simulink model "Mission__SimulatorModel"  (Simulink 10.1)
settings: Solver=ode8  StartTime=0.0  StopTime=100000  FixedStep=time_step  RelTol=1e-3
StartFcn:
  | % copyfile(char(CurrentFolder + "\3DModels\" + string(MODELO_3D)), char(CurrentFolder + "\" + string(MODELO_3D)));
StopFcn:
  | % delete(MODELO_3D)
values from neighbouring files (symbols this model uses):
  Aileron_Trim = -deltaa_trim_med/2    [Trim_ArcDME2.m]
  Elevator_Trim = deltae_trim_med    [Trim_ArcDME2.m]    (also in Trim_ClimbXZ2.m; Trim_CruiseThetaXZ2.m)
  Engine_Trim = lever_trim_med    [Trim_ArcDME2.m]    (also in Trim_ClimbXZ2.m; Trim_CruiseThetaXZ2.m)
  phi_ini = phi_ini_trim_med    [Trim_ArcDME2.m]
  u_ini = u_ini_trim_med    [Trim_ArcDME2.m]    (also in Trim_ClimbXZ2.m; Trim_CruiseThetaXZ2.m)
  v_ini = v_ini_trim2    [Trim_ArcDME2.m]    (also in Trim_ClimbXZ2.m; Trim_CruiseThetaXZ2.m)
  w_ini = -UVW_aux(3)    [Trim_ArcDME2.m]    (also in Trim_ClimbXZ2.m = -UVW_aux2(3) + UVW_aux1(3); Trim_CruiseThetaXZ2.m)
undefined symbols (not defined in the file or in its folder): AoA_alpha_max, AoA_beta_max, b, c, cargo_mass, CD0_interp, CD_ajus_coef, CD_beta_interp, CD_mach_reg, CDde, CDflap, CDgear, CDi, CDsb, CDsp, CL_ajus_coef, CL_alpha_interp, CL_alpha_reg, Clb, Clda_interp, CLde, Cldr, Clp, Clr, Cm0, Cm_alpha, Cmadot, Cmde_ajus_coef, Cmde_interp, Cmq, Cnb, Cndr, Cnr, Coef_Aileron_Beta, Coef_Aileron_Phi, Coef_Aileron_Rudder, Coef_Elevator_Alpha, Coef_Rudder_Aileron, Coef_Rudder_Beta, CYb, dCLflap, dfuel, dfuel0, e0_0, e1_0, e2_0, e3_0, fuel, fuel_density, fuel_max, g, GeoDate_Ap, GeoDate_Day, GeoDate_LatLongElv, GeoDate_Time, Ixx, Ixz, Iyy, Izz, kCDge_interp ... (+35)
libraries: aerolibconvert2 x17, aerolibutil x14, dsppolyfun x7, aerolibactuator x5, sharedtransform x4, robotcorelib x4, simulink x3, visionstatistics x3, vrlib x2, aerolibasang x1
(part 2 of 3)

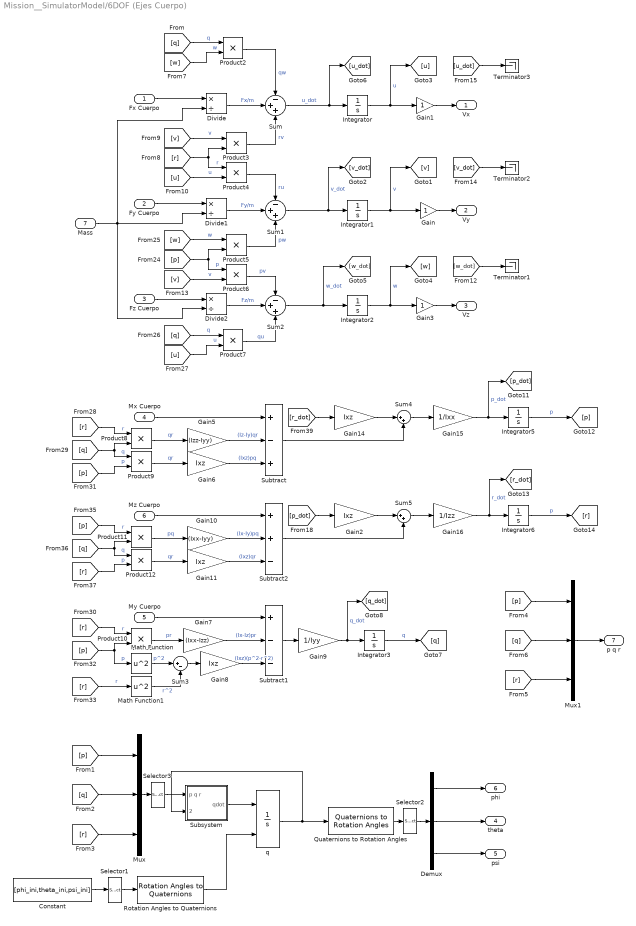
== system Mission__SimulatorModel/6DOF (Ejes Cuerpo) ==
  Fx Cuerpo : Inport
  Fy Cuerpo : Inport  Port=2
  Fz Cuerpo : Inport  Port=3
  Mx Cuerpo : Inport  Port=4
  My Cuerpo : Inport  Port=5
  Mz Cuerpo : Inport  Port=6
  Mass : Inport  Port=7
  Constant : Constant  Value=[phi_ini,theta_ini,psi_ini]
  Demux : Demux  Outputs=3
  Divide : Product  Inputs=*/
  Divide1 : Product  Inputs=*/
  Divide2 : Product  Inputs=*/
  Gain : Gain
  Gain1 : Gain
  Gain10 : Gain  Gain=(Ixx-Iyy)
  Gain{2,6,8,11,14} (5 alike) : Gain  Gain=Ixz
  Gain15 : Gain  Gain=1/Ixx
  Gain16 : Gain  Gain=1/Izz
  Gain3 : Gain
  Gain5 : Gain  Gain=(Izz-Iyy)
  Gain7 : Gain  Gain=(Ixx-Izz)
  Gain9 : Gain  Gain=1/Iyy
  Integrator : Integrator  InitialCondition=u_ini+0.000000000001
  Integrator1 : Integrator  InitialCondition=v_ini
  Integrator2 : Integrator  InitialCondition=w_ini
  Integrator3 : Integrator  InitialCondition=q_ini
  Integrator5 : Integrator  InitialCondition=p_ini
  Integrator6 : Integrator  InitialCondition=r_ini
  Math Function : Math  Operator=square  SaturateOnIntegerOverflow=on
  Math Function1 : Math  Operator=square  SaturateOnIntegerOverflow=on
  Mux : Mux  Inputs=3
  Mux1 : Mux  Inputs=3
  Product{2..12} (11 alike) : Product
  Quaternions to Rotation Angles : sharedtransform/Quaternions to Rotation Angles  rotationOrder=XYZ  aMode=aMode
      settings: SourceProductBaseCode=AE,PW,MT,VE,VP
  Rotation Angles to Quaternions : sharedtransform/Rotation Angles to Quaternions  rotationOrder=XYZ  aMode=aMode
      settings: SourceProductBaseCode=AE,PW,MT,VE,VP
  Selector1 : Selector  InputPortWidth=3  IndexOptions=Index vector (dialog)  Indices=[3 2 1]  OutputSizes=1
  Selector2 : Selector  InputPortWidth=3  IndexOptions=Index vector (dialog)  Indices=[3 2 1]  OutputSizes=1
  Selector3 : Selector  InputPortWidth=3  IndexOptions=Index vector (dialog)  Indices=[3 2 1]  OutputSizes=1
  Subsystem : Subsystem
  Subtract : Sum  Inputs=+-+
  Subtract1 : Sum  Inputs=+--
  Subtract2 : Sum  Inputs=++-
  Sum : Sum  Inputs=-++
  Sum1 : Sum  Inputs=-++
  Sum2 : Sum  Inputs=-++
  Sum3 : Sum  Inputs=|+-
  Sum4 : Sum  Inputs=|++
  Sum5 : Sum  Inputs=|++
  Terminator1 : Terminator
  Terminator2 : Terminator
  Terminator3 : Terminator
  q : Integrator  InitialConditionSource=external  InitialCondition=[e0_0 e1_0 e2_0 e3_0]
  Vx : Outport
  Vy : Outport  Port=2
  Vz : Outport  Port=3
  theta : Outport  Port=4
  psi : Outport  Port=5
  phi : Outport  Port=6
  p q r : Outport  Port=7
  wires:
  Sum1/1 -> [v_dot], Integrator1/1  "v_dot"
  Gain15/1 -> [p_dot], Integrator5/1  "p_dot"
  Math Function1/1 -> Sum3/2  "r^2"
  Integrator1/1 -> [v], Gain/1  "v"
  [q] -> Product9/1, Product8/2  "q"
  Integrator2/1 -> Gain3/1, [w]  "w"
  Math Function/1 -> Sum3/1  "p^2"
  Product2/1 -> Sum/1  "qw"
  Sum/1 -> [u_dot], Integrator/1  "u_dot"
  Product4/1 -> Sum1/1  "ru"
  [u] -> Product4/2  "u"
  [r] -> Product8/1  "r"
  [q] -> Product7/1  "q"
  Sum3/1 -> Gain8/1
  Fx Cuerpo/1 -> Divide/1
  Fz Cuerpo/1 -> Divide2/1
  Product12/1 -> Gain11/1  "qr"
  Subtract1/1 -> Gain9/1
  [u] -> Product7/2  "u"
  Subtract/1 -> Sum4/2
  [w] -> Product5/1  "w"
  [r] -> Product4/1, Product3/2  "r"
  Product7/1 -> Sum2/3  "qu"
  Gain6/1 -> Subtract/3  "(Ixz)pq"
  [p] -> Math Function/1, Product10/2  "p"
  Gain9/1 -> [q_dot], Integrator3/1  "q_dot"
  Sum2/1 -> [w_dot], Integrator2/1  "w_dot"
  Product5/1 -> Sum1/3  "pw"
  Gain7/1 -> Subtract1/2  "(Ix-Iz)pr"
  Integrator5/1 -> [p]  "p"
  Divide/1 -> Sum/2  "Fx/m"
  Gain10/1 -> Subtract2/2  "(Ix-Iy)pq"
  [r] -> Math Function1/1  "r"
  Fy Cuerpo/1 -> Divide1/1
  [p] -> Product5/2, Product6/1  "p"
  [p] -> Product9/2  "p"
  [r_dot] -> Gain14/1
  Product11/1 -> Gain10/1  "pq"
  [v] -> Product3/1  "v"
  Subtract2/1 -> Sum5/2
  Gain8/1 -> Subtract1/3  "(Ixz)(p^2-r^2)"
  Gain11/1 -> Subtract2/3  "(Ixz)qr"
  [r] -> Product12/2  "p"
  [w] -> Product2/2  "w"
  [p] -> Product11/1  "r"
  Product8/1 -> Gain5/1  "qr"
  Integrator3/1 -> [q]  "q"
  [q] -> Product11/2, Product12/1  "q"
  [r] -> Product10/1  "r"
  Integrator/1 -> Gain1/1, [u]  "u"
  Divide2/1 -> Sum2/2  "Fz/m"
  Gain14/1 -> Sum4/1
  [v] -> Product6/2  "v"
  Product9/1 -> Gain6/1  "qr"
  Divide1/1 -> Sum1/2  "Fy/m"
  Sum4/1 -> Gain15/1
  [q] -> Product2/1  "q"
  Gain5/1 -> Subtract/2  "(Iz-Iy)qr"
  Product3/1 -> Sum/3  "rv"
  Product6/1 -> Sum2/1  "pv"
  Product10/1 -> Gain7/1  "pr"
  Mz Cuerpo/1 -> Subtract2/1
  Mx Cuerpo/1 -> Subtract/1
  My Cuerpo/1 -> Subtract1/1
  [p] -> Mux/1
  [q] -> Mux/2
  [r] -> Mux/3
  Subsystem/1(qdot) -> q/1
  Constant/1 -> Selector1/1
  q/1 -> Subsystem/2(q0 q1 q2 q3), Quaternions to Rotation Angles/1
  Quaternions to Rotation Angles/1 -> Selector2/1
  Demux/2 -> theta/1
  Mux1/1 -> p q r/1
  [q] -> Mux1/2
  [p] -> Mux1/1
  [r] -> Mux1/3
  [w_dot] -> Terminator1/1
  [v_dot] -> Terminator2/1
  [u_dot] -> Terminator3/1
  Demux/1 -> phi/1
  Selector1/1 -> Rotation Angles to Quaternions/1
  Selector2/1 -> Demux/1
  Selector3/1 -> Subsystem/1(p q r)
  Gain16/1 -> [r_dot], Integrator6/1  "r_dot"
  [p_dot] -> Gain2/1
  Gain2/1 -> Sum5/1
  Sum5/1 -> Gain16/1
  Integrator6/1 -> [r]  "p"
  Mass/1 -> Divide/2, Divide2/2, Divide1/2
  Demux/3 -> psi/1
  Gain/1 -> Vy/1
  Gain1/1 -> Vx/1
  Gain3/1 -> Vz/1
  Rotation Angles to Quaternions/1 -> q/2
  Mux/1 -> Selector3/1

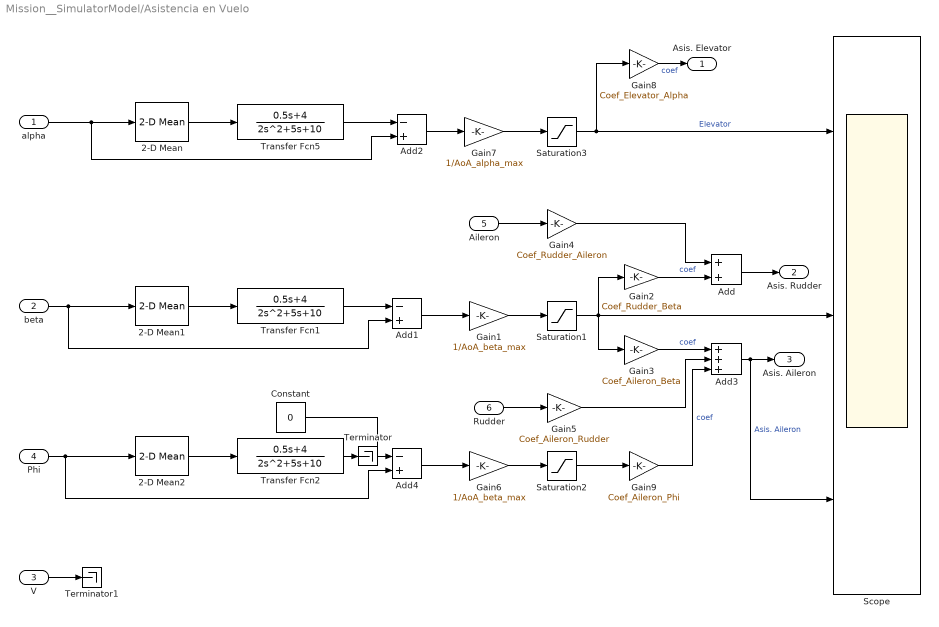
== system Mission__SimulatorModel/Asistencia en Vuelo ==
  alpha : Inport
  beta : Inport  Port=2
  V : Inport  Port=3
  Phi : Inport  Port=4
  Aileron : Inport  Port=5
  Rudder : Inport  Port=6
  2-D Mean : visionstatistics/2-D Mean  run=on  reset_popup=None  directionMode=Specified dimension  dimension=25  treatSBRowAsCol=on  outputLastDataTypeStr=Inherit: Same as accumulator  accumMode=Binary point scaling  accumWordLength=32  accumFracLength=0  accumLastDataTypeStr=fixdt([],32,0)  roiEnable=off  roiType=Rectangles  roiPortion=Entire ROI  roiOutput=Individual statistics for each ROI  roiFlag=off  roundingMode=Floor  overflowMode=off  accumDataTypeStr=fixdt([],32,0)  outputDataTypeStr=Inherit: Same as accumulator  outputMin=[]  outputMax=[]
      settings: SourceProductBaseCode=VP
  2-D Mean1 : visionstatistics/2-D Mean  run=on  reset_popup=None  directionMode=Specified dimension  dimension=25  treatSBRowAsCol=on  outputLastDataTypeStr=Inherit: Same as accumulator  accumMode=Binary point scaling  accumWordLength=32  accumFracLength=0  accumLastDataTypeStr=fixdt([],32,0)  roiEnable=off  roiType=Rectangles  roiPortion=Entire ROI  roiOutput=Individual statistics for each ROI  roiFlag=off  roundingMode=Floor  overflowMode=off  accumDataTypeStr=fixdt([],32,0)  outputDataTypeStr=Inherit: Same as accumulator  outputMin=[]  outputMax=[]
      settings: SourceProductBaseCode=VP
  2-D Mean2 : visionstatistics/2-D Mean  run=on  reset_popup=None  directionMode=Specified dimension  dimension=300  treatSBRowAsCol=on  outputLastDataTypeStr=Inherit: Same as accumulator  accumMode=Binary point scaling  accumWordLength=32  accumFracLength=0  accumLastDataTypeStr=fixdt([],32,0)  roiEnable=off  roiType=Rectangles  roiPortion=Entire ROI  roiOutput=Individual statistics for each ROI  roiFlag=off  roundingMode=Floor  overflowMode=off  accumDataTypeStr=fixdt([],32,0)  outputDataTypeStr=Inherit: Same as accumulator  outputMin=[]  outputMax=[]
      settings: SourceProductBaseCode=VP
  Add : Sum
  Add1 : Sum  Inputs=-+
  Add2 : Sum  Inputs=-+
  Add3 : Sum  Inputs=+++
  Add4 : Sum  Inputs=-+
  Constant : Constant  Value=0
  Gain1 : Gain  Gain=1/AoA_beta_max
  Gain2 : Gain  Gain=Coef_Rudder_Beta
  Gain3 : Gain  Gain=Coef_Aileron_Beta
  Gain4 : Gain  Gain=Coef_Rudder_Aileron
  Gain5 : Gain  Gain=Coef_Aileron_Rudder
  Gain6 : Gain  Gain=1/AoA_beta_max
  Gain7 : Gain  Gain=1/AoA_alpha_max
  Gain8 : Gain  Gain=Coef_Elevator_Alpha
  Gain9 : Gain  Gain=Coef_Aileron_Phi
  Saturation1 : Saturate  UpperLimit=1  LowerLimit=-1
  Saturation2 : Saturate  UpperLimit=1  LowerLimit=-1
  Saturation3 : Saturate  UpperLimit=1  LowerLimit=-1
  Scope : Scope  NumInputPorts=3
  Terminator : Terminator
  Terminator1 : Terminator
  Transfer Fcn1 : TransferFcn  Numerator=[0.5 4]  Denominator=[2 5 10]
  Transfer Fcn2 : TransferFcn  Numerator=[0.5 4]  Denominator=[2 5 10]
  Transfer Fcn5 : TransferFcn  Numerator=[0.5 4]  Denominator=[2 5 10]
  Asis. Elevator : Outport
  Asis. Rudder : Outport  Port=2
  Asis. Aileron : Outport  Port=3
  wires:
  Gain8/1 -> Asis. Elevator/1  "coef"
  Gain7/1 -> Saturation3/1
  Add2/1 -> Gain7/1
  alpha/1 -> 2-D Mean/1, Add2/2
  Saturation3/1 -> Gain8/1, Scope/1  "Elevator"
  Transfer Fcn5/1 -> Add2/1
  2-D Mean1/1 -> Transfer Fcn1/1
  Transfer Fcn1/1 -> Add1/1
  Saturation1/1 -> Gain2/1, Scope/2, Gain3/1
  beta/1 -> Add1/2, 2-D Mean1/1
  Add1/1 -> Gain1/1
  Gain1/1 -> Saturation1/1
  Gain2/1 -> Add/2  "coef"
  Aileron/1 -> Gain4/1
  Gain4/1 -> Add/1
  Rudder/1 -> Gain5/1
  Gain5/1 -> Add3/2
  Add3/1 -> Asis. Aileron/1, Scope/3  "Asis. Aileron"
  Gain3/1 -> Add3/1  "coef"
  Add4/1 -> Gain6/1
  Phi/1 -> 2-D Mean2/1, Add4/2
  2-D Mean2/1 -> Transfer Fcn2/1
  Gain6/1 -> Saturation2/1
  Saturation2/1 -> Gain9/1
  Gain9/1 -> Add3/3  "coef"
  Transfer Fcn2/1 -> Terminator/1
  Constant/1 -> Add4/1
  Add/1 -> Asis. Rudder/1
  2-D Mean/1 -> Transfer Fcn5/1
  V/1 -> Terminator1/1

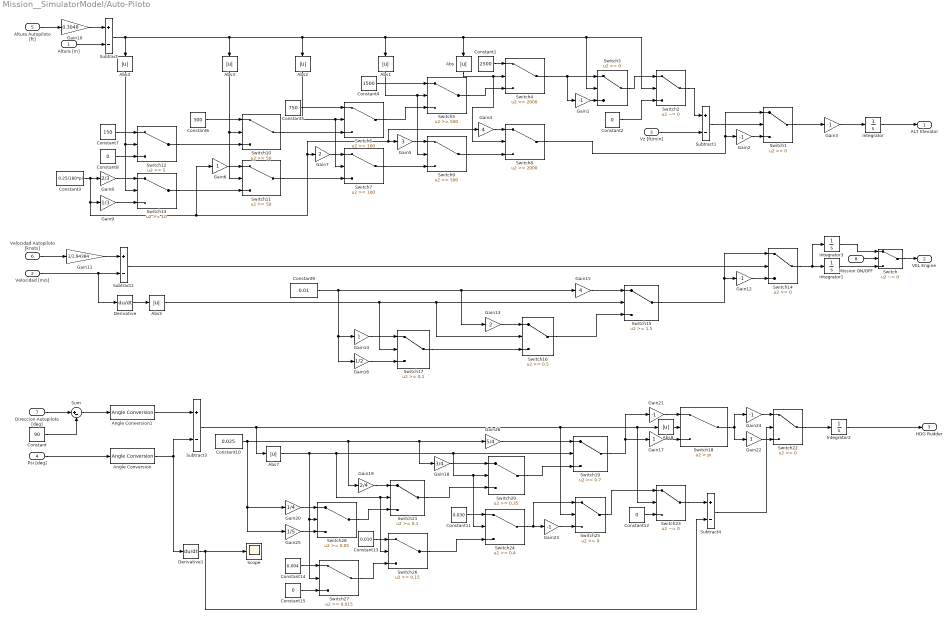
== system Mission__SimulatorModel/Auto-Piloto ==
  Altura [m] : Inport
  Velocidad [m/s] : Inport  Port=2
  Vz [ft/min] : Inport  Port=3
  Psi [deg] : Inport  Port=4
  Altura Autopiloto [ft] : Inport  Port=5
  Velocidad Autopiloto [knots] : Inport  Port=6
  Direccion Autopiloto [deg] : Inport  Port=7
  Mission ON/OFF : Inport  Port=8
  Abs{,1..5,7..8} (8 alike) : Abs
  Angle Conversion : aerolibconvert2/Angle Conversion  IU=deg  OU=rad
  Angle Conversion1 : aerolibconvert2/Angle Conversion  IU=deg  OU=rad
  Constant : Constant  Value=90
  Constant1 : Constant  Value=2500
  Constant10 : Constant  Value=0.025
  Constant11 : Constant  Value=0.030
  Constant{2,8,12,15} (4 alike) : Constant  Value=0
  Constant13 : Constant  Value=0.010
  Constant14 : Constant  Value=0.004
  Constant3 : Constant  Value=0.25/180*pi
  Constant4 : Constant  Value=1500
  Constant5 : Constant  Value=750
  Constant6 : Constant  Value=300
  Constant7 : Constant  Value=150
  Constant9 : Constant  Value=0.01
  Derivative : Derivative
  Derivative1 : Derivative
  Gain{1..3,12,21,23..24} (7 alike) : Gain  Gain=-1
  Gain10 : Gain  Gain=0.3048
  Gain11 : Gain  Gain=1/1.94384
  Gain13 : Gain  Gain=2
  Gain{6,14,17,22} (4 alike) : Gain
  Gain15 : Gain  Gain=4
  Gain16 : Gain  Gain=1/2
  Gain18 : Gain  Gain=3/4
  Gain19 : Gain  Gain=2/4
  Gain20 : Gain  Gain=1/4
  Gain25 : Gain  Gain=1/5
  Gain26 : Gain  Gain=5/4
  Gain4 : Gain  Gain=4
  Gain5 : Gain  Gain=3
  Gain7 : Gain  Gain=2
  Gain8 : Gain  Gain=2/3
  Gain9 : Gain  Gain=1/3
  Integrator : Integrator  LimitOutput=on  UpperSaturationLimit=0.4  LowerSaturationLimit=-0.4
  Integrator1 : Integrator  LimitOutput=on  UpperSaturationLimit=0.2  LowerSaturationLimit=-0.2
  Integrator2 : Integrator  LimitOutput=on  UpperSaturationLimit=0.14  LowerSaturationLimit=-0.14
  Integrator3 : Integrator  LimitOutput=on  UpperSaturationLimit=0.5  LowerSaturationLimit=-0.5
  Scope : Scope
  Subtract{,1..4} (5 alike) : Sum  Inputs=+-
  Sum : Sum  Inputs=|+-
  Switch : Switch  Criteria=u2 ~= 0
  Switch{1,3,14,22,25} (5 alike) : Switch
  Switch10 : Switch  Threshold=50
  Switch11 : Switch  Threshold=50
  Switch12 : Switch  Threshold=5
  Switch13 : Switch  Threshold=10
  Switch15 : Switch  Threshold=1.5
  Switch16 : Switch  Threshold=0.5
  Switch17 : Switch  Threshold=0.1
  Switch18 : Switch  Criteria=u2 > Threshold  Threshold=pi
  Switch19 : Switch  Threshold=0.7
  Switch2 : Switch  Criteria=u2 ~= 0
  Switch20 : Switch  Threshold=0.35
  Switch21 : Switch  Threshold=0.1
  Switch23 : Switch  Criteria=u2 ~= 0
  Switch24 : Switch  Threshold=0.4
  Switch26 : Switch  Threshold=0.15
  Switch27 : Switch  Threshold=0.015
  Switch28 : Switch  Threshold=0.05
  Switch4 : Switch  Threshold=2000
  Switch5 : Switch  Threshold=500
  Switch6 : Switch  Threshold=100
  Switch7 : Switch  Threshold=100
  Switch8 : Switch  Threshold=2000
  Switch9 : Switch  Threshold=500
  ALT Elevator : Outport
  VEL Engine : Outport  Port=2
  HDG Rudder : Outport  Port=3
  wires:
  Subtract/1 -> Switch3/2, Switch2/2, Abs/1, Abs1/1, Abs2/1, Abs3/1, Abs4/1
  Altura Autopiloto [ft]/1 -> Gain10/1
  Altura [m]/1 -> Subtract/2
  Subtract1/1 -> Switch1/2
  Vz [ft/min]/1 -> Subtract1/2
  Gain2/1 -> Switch1/3
  Switch1/1 -> Gain3/1
  Integrator/1 -> ALT Elevator/1
  Switch4/1 -> Switch3/1, Gain1/1
  Gain1/1 -> Switch3/3
  Switch3/1 -> Switch2/1
  Constant2/1 -> Switch2/3
  Switch2/1 -> Subtract1/1
  Gain3/1 -> Integrator/1
  Abs/1 -> Switch8/2, Switch4/2
  Constant1/1 -> Switch4/1
  Abs1/1 -> Switch9/2, Switch5/2
  Switch5/1 -> Switch4/3
  Constant4/1 -> Switch5/1
  Switch6/1 -> Switch5/3
  Constant5/1 -> Switch6/1
  Abs2/1 -> Switch7/2, Switch6/2
  Switch8/1 -> Switch1/1, Gain2/1
  Gain4/1 -> Switch8/1
  Switch9/1 -> Switch8/3
  Gain5/1 -> Switch9/1
  Constant3/1 -> Gain9/1, Gain6/1, Gain4/1, Gain5/1, Gain7/1, Gain8/1
  Gain6/1 -> Switch11/1
  Switch7/1 -> Switch9/3
  Switch10/1 -> Switch6/3
  Constant6/1 -> Switch10/1
  Switch12/1 -> Switch10/3
  Gain7/1 -> Switch7/1
  Switch11/1 -> Switch7/3
  Switch13/1 -> Switch11/3
  Constant7/1 -> Switch12/1
  Constant8/1 -> Switch12/3
  Gain8/1 -> Switch13/1
  Gain9/1 -> Switch13/3
  Abs3/1 -> Switch10/2, Switch11/2
  Abs4/1 -> Switch12/2, Switch13/2
  Gain10/1 -> Subtract/1
  Velocidad Autopiloto [knots]/1 -> Gain11/1
  Gain11/1 -> Subtract2/1
  Velocidad [m/s]/1 -> Derivative/1, Subtract2/2
  Subtract2/1 -> Switch14/2
  Switch14/1 -> Integrator3/1, Integrator1/1
  Gain12/1 -> Switch14/3
  Switch15/1 -> Switch14/1, Gain12/1
  Derivative/1 -> Abs5/1
  Abs5/1 -> Switch17/2, Switch16/2, Switch15/2
  Switch16/1 -> Switch15/3
  Constant9/1 -> Gain16/1, Gain14/1, Gain13/1, Gain15/1
  Gain13/1 -> Switch16/1
  Switch17/1 -> Switch16/3
  Gain15/1 -> Switch15/1
  Gain14/1 -> Switch17/1
  Gain16/1 -> Switch17/3
  Psi [deg]/1 -> Angle Conversion/1
  Sum/1 -> Angle Conversion1/1
  Direccion Autopiloto [deg]/1 -> Sum/1
  Constant/1 -> Sum/2
  Integrator2/1 -> HDG Rudder/1
  Gain17/1 -> Switch18/3
  Subtract3/1 -> Abs7/1, Switch25/2, Switch23/2, Abs8/1
  Derivative1/1 -> Subtract4/2, Scope/1
  Angle Conversion1/1 -> Subtract3/1
  Angle Conversion/1 -> Subtract3/2, Derivative1/1
  Switch19/1 -> Gain17/1, Gain21/1
  Switch20/1 -> Switch19/3
  Switch21/1 -> Switch20/3
  Abs7/1 -> Switch28/2, Switch27/2, Switch24/2, Switch20/2, Switch19/2, Switch26/2, Switch21/2
  Constant10/1 -> Gain25/1, Gain20/1, Gain18/1, Gain26/1, Gain19/1
  Gain18/1 -> Switch20/1
  Gain19/1 -> Switch21/1
  Gain21/1 -> Switch18/1
  Switch22/1 -> Integrator2/1
  Gain22/1 -> Switch22/3
  Switch23/1 -> Subtract4/1
  Subtract4/1 -> Switch22/2
  Constant12/1 -> Switch23/3
  Switch25/1 -> Switch23/1
  Gain23/1 -> Switch25/3
  Switch24/1 -> Switch25/1, Gain23/1
  Constant11/1 -> Switch24/1
  Switch26/1 -> Switch24/3
  Constant13/1 -> Switch26/1
  Constant14/1 -> Switch27/1
  Switch27/1 -> Switch26/3
  Constant15/1 -> Switch27/3
  Gain24/1 -> Switch22/1
  Switch28/1 -> Switch21/3
  Gain20/1 -> Switch28/1
  Gain25/1 -> Switch28/3
  Gain26/1 -> Switch19/1
  Switch18/1 -> Gain24/1, Gain22/1
  Abs8/1 -> Switch18/2
  Switch/1 -> VEL Engine/1
  Mission ON/OFF/1 -> Switch/2
  Integrator3/1 -> Switch/1
  Integrator1/1 -> Switch/3

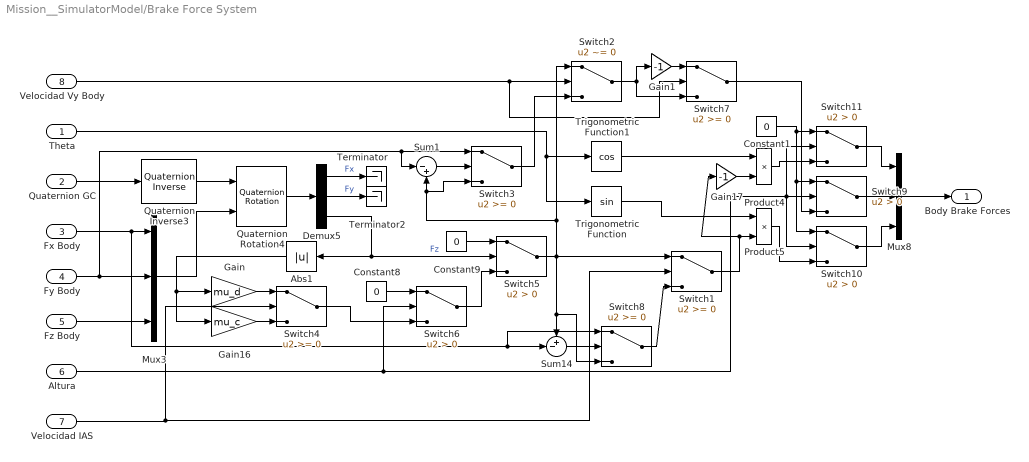
== system Mission__SimulatorModel/Brake Force System ==
  Theta : Inport
  Quaternion GC : Inport  Port=2
  Fx Body : Inport  Port=3
  Fy Body : Inport  Port=4
  Fz Body : Inport  Port=5
  Altura : Inport  Port=6
  Velocidad IAS : Inport  Port=7
  Velocidad Vy Body : Inport  Port=8
  Abs1 : Abs
  Constant1 : Constant  Value=0
  Constant8 : Constant  Value=0
  Constant9 : Constant  Value=0
  Demux5 : Demux  Outputs=3
  Gain : Gain  Gain=mu_d
  Gain1 : Gain  Gain=-1
  Gain16 : Gain  Gain=mu_c
  Gain17 : Gain  Gain=-1
  Mux3 : Mux  Inputs=3
  Mux8 : Mux  Inputs=3
  Product4 : Product
  Product5 : Product
  Quaternion Inverse3 : aerolibutil/Quaternion Inverse
  Quaternion Rotation4 : aerolibutil/Quaternion Rotation
  Sum1 : Sum  Inputs=|-+
  Sum14 : Sum  Inputs=+-|
  Switch{1,3..4,7..8} (5 alike) : Switch
  Switch{5..6,9..11} (5 alike) : Switch  Criteria=u2 > Threshold
  Switch2 : Switch  Criteria=u2 ~= 0
  Terminator : Terminator
  Terminator2 : Terminator
  Trigonometric Function : Trigonometry
  Trigonometric Function1 : Trigonometry  Operator=cos
  Body Brake Forces : Outport
  wires:
  Quaternion Rotation4/1 -> Demux5/1
  Quaternion Inverse3/1 -> Quaternion Rotation4/1
  Switch4/1 -> Switch6/3
  Mux3/1 -> Quaternion Rotation4/2
  Demux5/3 -> Switch5/2, Abs1/1  "Fz"
  Fz Body/1 -> Mux3/3
  Demux5/1 -> Terminator/1  "Fx"
  Fx Body/1 -> Switch8/1, Sum14/2, Mux3/1
  Trigonometric Function/1 -> Product5/1
  Theta/1 -> Trigonometric Function/1, Trigonometric Function1/1
  Sum14/1 -> Switch8/2
  Switch1/1 -> Gain17/1, Product5/2
  Constant9/1 -> Switch5/1
  Trigonometric Function1/1 -> Product4/1
  Fy Body/1 -> Switch3/1, Sum1/1, Mux3/2
  Gain17/1 -> Product4/2
  Switch5/1 -> Switch3/3, Sum1/2, Switch2/1, Sum14/1, Switch8/3, Switch1/1
  Gain/1 -> Switch4/1
  Mux8/1 -> Body Brake Forces/1
  Abs1/1 -> Gain16/1, Gain/1
  Constant8/1 -> Switch6/1
  Gain16/1 -> Switch4/3
  Switch6/1 -> Switch5/3
  Demux5/2 -> Terminator2/1  "Fy"
  Quaternion GC/1 -> Quaternion Inverse3/1
  Altura/1 -> Switch10/2, Switch11/2, Switch9/2, Switch6/2
  Velocidad IAS/1 -> Switch1/2, Switch4/2
  Switch8/1 -> Switch1/3
  Velocidad Vy Body/1 -> Switch7/2, Switch2/2
  Switch3/1 -> Switch2/3
  Sum1/1 -> Switch3/2
  Gain1/1 -> Switch7/1
  Switch2/1 -> Switch7/3, Gain1/1
  Switch9/1 -> Mux8/2
  Switch7/1 -> Switch9/3
  Constant1/1 -> Switch10/1, Switch9/1, Switch11/1
  Product5/1 -> Switch10/3
  Product4/1 -> Switch11/3
  Switch11/1 -> Mux8/1
  Switch10/1 -> Mux8/3

== system Mission__SimulatorModel/Engine Alert ==
  Engine : Inport
  Constant : Constant
  Constant1 : Constant  Value=0
  Constant6 : Constant  Value=-1
  Constant7 : Constant  Value=2
  Constant8 : Constant
  Gain : Gain  Gain=1/100
  Sum : Sum  Inputs=|-+
  Switch1 : Switch  Criteria=u2 > Threshold  Threshold=0.2
  Switch4 : Switch  Criteria=u2 > Threshold  Threshold=0.6
  Switch5 : Switch  Criteria=u2 > Threshold  Threshold=0.4
  Engine Indicator : Outport
  wires:
  Switch4/1 -> Switch5/1
  Constant8/1 -> Switch5/3
  Constant7/1 -> Switch4/3
  Constant6/1 -> Switch4/1
  Constant1/1 -> Switch1/3
  Switch5/1 -> Switch1/1
  Engine/1 -> Gain/1
  Constant/1 -> Sum/2
  Sum/1 -> Switch5/2, Switch1/2, Switch4/2
  Switch1/1 -> Engine Indicator/1
  Gain/1 -> Sum/1

== system Mission__SimulatorModel/Fuel Alert ==
  Fuel Capacity : Inport
  Constant6 : Constant  Value=-1
  Constant7 : Constant  Value=0
  Constant8 : Constant
  Switch4 : Switch  Criteria=u2 > Threshold
  Switch5 : Switch  Criteria=u2 > Threshold  Threshold=0.4
  Lamp Indicator : Outport
  wires:
  Constant6/1 -> Switch4/1
  Fuel Capacity/1 -> Switch5/2, Switch4/2
  Constant7/1 -> Switch4/3
  Constant8/1 -> Switch5/3
  Switch4/1 -> Switch5/1
  Switch5/1 -> Lamp Indicator/1

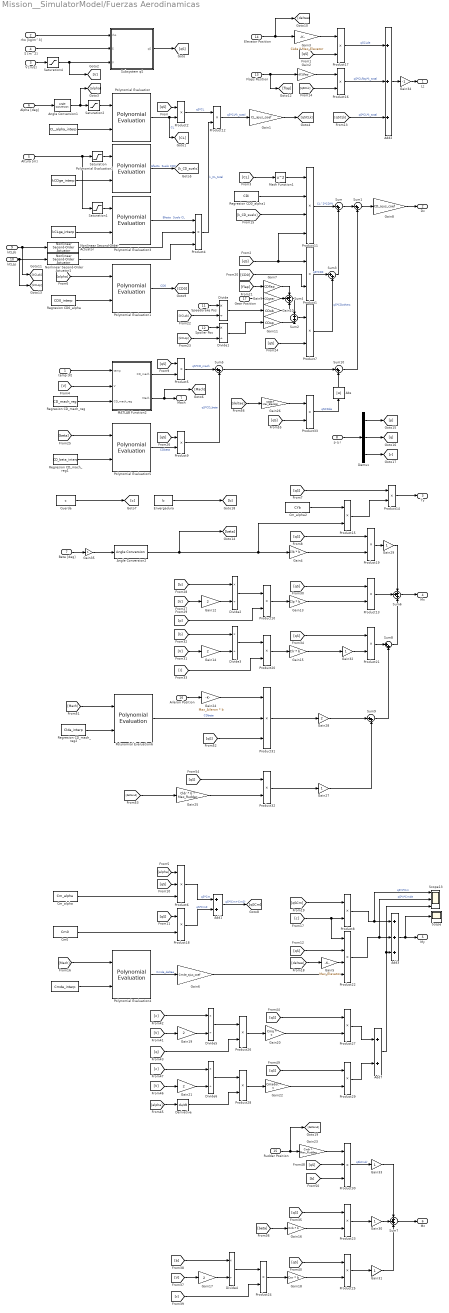
== system Mission__SimulatorModel/Fuerzas Aerodinamicas ==
  temp [K] : Inport
  rho [kg/m^3] : Inport  Port=2
  V [m/s] : Inport  Port=3
  S [m^2] : Inport  Port=4
  Altura [m] : Inport  Port=5
  Alpha [deg] : Inport  Port=6
  Beta [deg] : Inport  Port=7
  p q r : Inport  Port=8
  kCLsb : Inport  Port=9
  kCLsp : Inport  Port=10
  Speedbrake Pos : Inport  Port=11
  Spoiler Pos : Inport  Port=12
  Flaps Position : Inport  Port=13
  Elevator Position : Inport  Port=14
  Rudder Position : Inport  Port=15
  Aileron Position : Inport  Port=16
  Gear Position : Inport  Port=17
  " " : Constant  Value=kCLge_interp
  "  " : Constant  Value=kCDge_interp
  "   " : Constant  Value=CL_alpha_interp
  "    " : Constant  Value=Cmde_interp
  " Cm0" : Constant  Value=Cm0
  " Cm_alpha" : Constant  Value=Cm_alpha
  " Cm_alpha2" : Constant  Value=CYb
  Abs : Abs
  Add1 : Sum
  Add2 : Sum  Inputs=+++
  Add3 : Sum  Inputs=+++
  Add7 : Sum
  Angle Conversion1 : aerolibconvert2/Angle Conversion  IU=deg  OU=rad
  Angle Conversion2 : aerolibconvert2/Angle Conversion  IU=deg  OU=rad
  Cuerda : Constant  Value=c
  Demux : Demux  Outputs=3
  Derivative : Derivative
  Divide{,1..6} (7 alike) : Product  Inputs=*/
  Envergadura : Constant  Value=b
  Gain1 : Gain  Gain=CL_ajus_coef
  Gain10 : Gain  Gain=CDsb
  Gain11 : Gain  Gain=CDsp
  Gain{12,14,17,19,21,28} (6 alike) : Gain  Gain=2
  Gain13 : Gain  Gain=Clp * b
  Gain15 : Gain  Gain=Clr * b
  Gain16 : Gain  Gain=Cnb * b
  Gain18 : Gain  Gain=Cnr * b
  Gain2 : Gain  Gain=dCLflap
  Gain20 : Gain  Gain=Cmq * c
  Gain22 : Gain  Gain=Cmadot * c
  Gain23 : Gain  Gain=Cndr * Max_Rudder
  Gain24 : Gain  Gain=Max_Aileron * b
  Gain25 : Gain  Gain=Cldr * b * Max_Rudder
  Gain26 : Gain  Gain=CDde * Max_Elevator
  Gain{27,29..33,35} (7 alike) : Gain
  Gain3 : Gain  Gain=CLde * Max_Elevator
  Gain34 : Gain  Gain=-1
  Gain4 : Gain  Gain=Clb * b
  Gain5 : Gain  Gain=Max_Elevator
  Gain6 : Gain  Gain=Cmde_ajus_coef
  Gain7 : Gain  Gain=CDflap
  Gain8 : Gain  Gain=CD_ajus_coef
  Gain9 : Gain  Gain=CDgear
  MATLAB Function2 : MATLAB Function  TreatAsAtomicUnit=on
  Math Function1 : Math  Operator=square  SaturateOnIntegerOverflow=on
  Nonlinear Second-Order Actuator : aerolibactuator/Nonlinear Second-Order Actuator  wn_fin=4  z_fin=1  fin_max=inf  fin_min=-inf  fin_maxrate=500*pi/180/1.9/2  fin_act_0=1  fin_act_vel=0
      settings: SourceProductBaseCode=AE
  Nonlinear Second-Order Actuator1 : aerolibactuator/Nonlinear Second-Order Actuator  wn_fin=4  z_fin=1  fin_max=inf  fin_min=-inf  fin_maxrate=500*pi/180/1.9/2  fin_act_0=1  fin_act_vel=0
      settings: SourceProductBaseCode=AE
  Polynomial Evaluation{,1..6} (7 alike) : dsppolyfun/Polynomial Evaluation  useConstCoeffs=off  constCoeffs=[5 4 3 2 1]
      settings: SourceProductBaseCode=DS
  Product{1..2,5,7..10,12..21,23..29,32..33} (26 alike) : Product
  Product11 : Product  Inputs=4
  Product22 : Product  Inputs=4
  Product{4,6,30..31} (4 alike) : Product  Inputs=3
  Regresion CD0_alpha : Constant  Value=CD0_interp
  Regresion CD0_alpha1 : Constant  Value=CDi
  Regresion CD_mach_reg : Constant  Value=CD_mach_reg
  Regresion CD_mach_reg1 : Constant  Value=CD_beta_interp
  Regresion CD_mach_reg2 : Constant  Value=Clda_interp
  Saturation : Saturate  UpperLimit=max_h_kCDge  LowerLimit=min_h_kCDge
  Saturation1 : Saturate  UpperLimit=max_h_kCLge  LowerLimit=min_h_kCLge
  Saturation2 : Saturate  UpperLimit=max(CL_alpha_reg(:,1))+(10/180*pi)  LowerLimit=min(CL_alpha_reg(:,1))-(5/180*pi)
  Saturation4 : Saturate  UpperLimit=inf  LowerLimit=0
  Scope : Scope
  Scope13 : Scope  NumInputPorts=3
  Subsystem qS : Subsystem
  Sum{,1,3,5,8..10} (7 alike) : Sum  Inputs=|++
  Sum2 : Sum
  Sum4 : Sum  Inputs=+++
  Sum6 : Sum  Inputs=+++
  Sum7 : Sum  Inputs=+++
  Lz : Outport
  Dx : Outport  Port=2
  Yy : Outport  Port=3
  Mx : Outport  Port=4
  My : Outport  Port=5
  Mz : Outport  Port=6
  Mach : Outport  Port=7
  wires:
  MATLAB Function2/1(CD_mach) -> Product5/2
  Polynomial Evaluation/1 -> [CL], Product2/2  "CL"
  Regresion CD0_alpha/1 -> Polynomial Evaluation1/2
  V [m/s]/1 -> Saturation4/1
  Product11/1 -> Sum/1  "CL^2*CDi*k"
  Sum/1 -> Sum1/1
  Regresion CD_mach_reg/1 -> MATLAB Function2/3(CD_mach_reg)
  temp [K]/1 -> MATLAB Function2/1(temp)
  MATLAB Function2/2(Mach) -> [Mach], Mach/1
  " Cm_alpha"/1 -> Product6/3
  Sum1/1 -> Gain8/1
  Angle Conversion1/1 -> [alpha], Saturation2/1
  Alpha [deg]/1 -> Angle Conversion1/1
  "   "/1 -> Polynomial Evaluation/2
  "  "/1 -> Polynomial Evaluation2/2
  Altura [m]/1 -> Saturation1/1, Saturation/1
  Saturation/1 -> Polynomial Evaluation2/1
  " "/1 -> Polynomial Evaluation3/2
  Saturation1/1 -> Polynomial Evaluation3/1
  Polynomial Evaluation3/1 -> Product4/1  "Efecto  Suelo CL"
  Product12/1 -> Gain1/1  "qS*CL*k_total"
  Product2/1 -> Product12/1  "qS*CL"
  Product4/1 -> Product12/2  "k_CL_total"
  kCLsp/1 -> Nonlinear Second-Order Actuator1/1, [kCLsp]
  Regresion CD0_alpha1/1 -> Product11/2
  Polynomial Evaluation2/1 -> [k_CD_suelo]  "Efecto  Suelo CD0"
  Product14/1 -> Yy/1
  Beta [deg]/1 -> Gain35/1
  " Cm_alpha2"/1 -> Product15/1
  Product15/1 -> Product14/2
  Add2/1 -> Gain34/1
  Product16/1 -> Add2/2  "qS*CLflap*k_total"
  Gain2/1 -> Product16/1
  Flaps Position/1 -> [flap], Gain2/1
  Product17/1 -> Add2/1  "qSCLde"
  Add1/1 -> [qSCm]  "qS*(Cm+Cm0)"
  " Cm0"/1 -> Product18/2
  Product18/1 -> Add1/2  "qS*Cm0"
  Product6/1 -> Add1/1  "qS*Cm"
  Gain4/1 -> Product19/2
  "    "/1 -> Polynomial Evaluation4/2
  Polynomial Evaluation4/1 -> Gain6/1  "Cmde_deltae"
  Gain6/1 -> Product22/4
  Add3/1 -> Scope/1, My/1
  Gain3/1 -> Product17/1
  Gain5/1 -> Product22/3
  Elevator Position/1 -> [deltae], Gain3/1
  Product22/1 -> Scope13/2, Add3/2  "qS*c*Cmde"
  Product8/1 -> Scope13/1, Add3/1  "qS*c*Cm"
  Gain8/1 -> Dx/1
  Subsystem qS/1(qS) -> [qS]
  rho [kg/m^3]/1 -> Subsystem qS/1(rho)
  S [m^2]/1 -> Subsystem qS/2(S)
  [qS] -> Product2/1
  [qS] -> Product17/2
  [alpha] -> Polynomial Evaluation1/1
  [qS] -> Product14/1
  [qS] -> Product19/1
  [qS] -> Product5/1
  [qS] -> Product6/2
  [qS] -> Product18/1
  [qS] -> Product22/2
  [qSCLk] -> Product16/2
  [k_CD_suelo] -> Product11/3
  [Mach] -> Polynomial Evaluation4/1
  Cuerda/1 -> [c]
  [c] -> Product22/1, Product8/2
  [qSCm] -> Product8/1
  Polynomial Evaluation1/1 -> [CD0]  "CD0"
  [deltae] -> Gain5/1
  Gain1/1 -> [qSCLk]
  [qSCLk] -> Add2/3  "qS*CL*k_total"
  [qS] -> Product11/4, Product1/1
  Math Function1/1 -> Product11/1
  kCLsb/1 -> Nonlinear Second-Order Actuator/1, [kCLsb]
  [CL] -> Math Function1/1
  Angle Conversion2/1 -> [beta], Product15/2, Gain4/1
  [flap] -> Gain7/1
  Gear Position/1 -> Gain9/1
  Speedbrake Pos/1 -> Divide/1
  Spoiler Pos/1 -> Divide1/1
  Divide1/1 -> Gain11/1
  [kCLsp] -> Divide1/2
  [kCLsb] -> Divide/2
  Divide/1 -> Gain10/1
  [CD0] -> Product1/2
  Gain9/1 -> Sum4/2
  Gain7/1 -> Sum4/1
  Gain10/1 -> Sum4/3
  Sum2/1 -> Product7/1
  Sum4/1 -> Sum2/1
  Gain11/1 -> Sum2/2
  [qS] -> Product7/2
  Product7/1 -> Sum3/2  "qS*CDothers"
  Product1/1 -> Sum3/1  "qS*CD0"
  Sum3/1 -> Sum/2
  [beta] -> Polynomial Evaluation5/1
  Regresion CD_mach_reg1/1 -> Polynomial Evaluation5/2
  Polynomial Evaluation5/1 -> Product9/2  "CDbeta"
  [qS] -> Product9/1
  Product9/1 -> Sum5/2  "qS*CD_beta"
  Product5/1 -> Sum5/1  "qS*CD_mach"
  [V] -> MATLAB Function2/2(V)
  p q r/1 -> Demux/1
  Demux/1 -> [p]
  Demux/2 -> [q]
  Demux/3 -> [r]
  Envergadura/1 -> [b]
  [V] -> Gain12/1
  Gain12/1 -> Divide2/2
  [b] -> Divide2/1
  Divide2/1 -> Product10/1
  Product10/1 -> Gain13/1
  [qS] -> Product13/1
  Gain13/1 -> Product13/2
  Product19/1 -> Gain29/1
  Gain15/1 -> Gain32/1
  [qS] -> Product21/1
  Product20/1 -> Gain15/1
  Divide3/1 -> Product20/1
  [b] -> Divide3/1
  Gain14/1 -> Divide3/2
  [V] -> Gain14/1
  [beta] -> Gain16/1
  [qS] -> Product23/1
  Gain16/1 -> Product23/2
  [V] -> Gain17/1
  Gain17/1 -> Divide4/2
  [b] -> Divide4/1
  Divide4/1 -> Product24/1
  [r] -> Product24/2
  Product24/1 -> Gain18/1
  [qS] -> Product25/1
  Gain18/1 -> Product25/2
  Gain20/1 -> Product27/2
  [qS] -> Product27/1
  Product26/1 -> Gain20/1
  [q] -> Product26/2
  Divide5/1 -> Product26/1
  [c] -> Divide5/1
  Gain19/1 -> Divide5/2
  [V] -> Gain19/1
  [alpha] -> Derivative/1
  [V] -> Gain21/1
  Gain21/1 -> Divide6/2
  [c] -> Divide6/1
  Divide6/1 -> Product28/1
  Derivative/1 -> Product28/2
  Product28/1 -> Gain22/1
  [qS] -> Product29/1
  Gain22/1 -> Product29/2
  Product29/1 -> Add7/2
  [qS] -> Product30/2
  Gain23/1 -> Product30/1
  [b] -> Product30/3
  Product27/1 -> Add7/1
  Add7/1 -> Scope13/3, Add3/3
  Rudder Position/1 -> [deltarud], Gain23/1
  Product30/1 -> Gain33/1  "qSbCndr"
  Product23/1 -> Gain30/1
  Product25/1 -> Gain31/1
  Regresion CD_mach_reg2/1 -> Polynomial Evaluation6/2
  [Mach] -> Polynomial Evaluation6/1
  Aileron Position/1 -> Gain24/1
  [qS] -> Product31/3
  Gain24/1 -> Product31/1
  Polynomial Evaluation6/1 -> Product31/2  "CDbeta"
  Sum8/1 -> Sum6/3
  [qS] -> Product32/1
  Gain25/1 -> Product32/2
  [deltarud] -> Gain25/1
  Product31/1 -> Gain28/1
  Product32/1 -> Gain27/1
  Product33/1 -> Abs/1  "qSCDde"
  [qS] -> Product33/2
  Gain26/1 -> Product33/1
  [deltae] -> Gain26/1
  Sum10/1 -> Sum1/2
  Sum5/1 -> Sum10/1
  Saturation2/1 -> Polynomial Evaluation/1
  [alpha] -> Product6/1
  Gain27/1 -> Sum9/2
  Gain28/1 -> Sum9/1
  Gain29/1 -> Sum6/1
  [p] -> Product10/2
  [r] -> Product20/2
  Gain30/1 -> Sum7/2
  Gain31/1 -> Sum7/3
  Gain32/1 -> Product21/2
  Nonlinear Second-Order Actuator/1 -> Product4/2
  Nonlinear Second-Order Actuator1/1 -> Product4/3
  Gain33/1 -> Sum7/1
  Sum7/1 -> Mz/1
  Saturation4/1 -> [V], Subsystem qS/3(V)
  Abs/1 -> Sum10/2
  Gain35/1 -> Angle Conversion2/1
  Product13/1 -> Sum6/2
  Product21/1 -> Sum8/1
  Sum9/1 -> Sum8/2
  Gain34/1 -> Lz/1
  Sum6/1 -> Mx/1

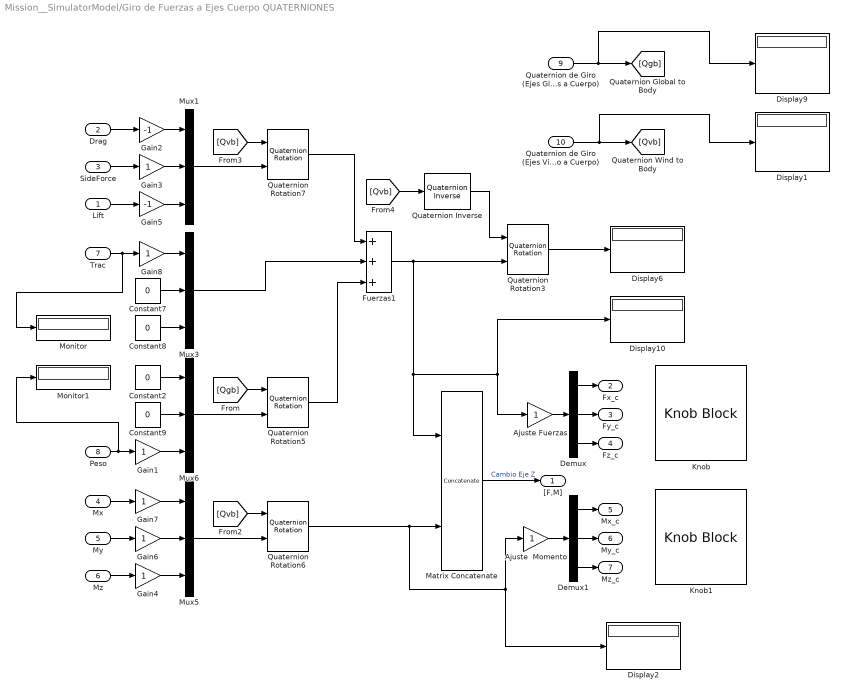
== system Mission__SimulatorModel/Giro de Fuerzas a Ejes Cuerpo QUATERNIONES ==
  Lift : Inport
  Drag : Inport  Port=2
  SideForce : Inport  Port=3
  Mx : Inport  Port=4
  My : Inport  Port=5
  Mz : Inport  Port=6
  Trac : Inport  Port=7
  Peso : Inport  Port=8
  Quaternion de Giro (Ejes Globales a Cuerpo) : Inport  Port=9
  Quaternion de Giro (Ejes Viento a Cuerpo) : Inport  Port=10
  Ajuste Fuerzas : Gain
  Ajuste  Momento : Gain
  Constant{2,7..9} (4 alike) : Constant  Value=0
  Demux : Demux  Outputs=3
  Demux1 : Demux  Outputs=3
  Display{1..2,6,9..10} (5 alike) : Display
  Fuerzas1 : Sum  Inputs=+++
  Gain{1,3..4,6..8} (6 alike) : Gain
  Gain2 : Gain  Gain=-1
  Gain5 : Gain  Gain=-1
  Knob : KnobBlock  LabelPosition=Hide  ScaleMin=0.01  ScaleMax=1
  Knob1 : KnobBlock  LabelPosition=Hide  ScaleMin=0.1  ScaleMax=4
  Matrix Concatenate : Concatenate  Mode=Multidimensional array  ConcatenateDimension=2
  Monitor : Display
  Monitor1 : Display
  Mux{1,3,5..6} (4 alike) : Mux  Inputs=3
  Quaternion Inverse : aerolibutil/Quaternion Inverse
  Quaternion Rotation{3,5..7} (4 alike) : aerolibutil/Quaternion Rotation
  "[F,M]" : Outport
  Fx_c : Outport  Port=2
  Fy_c : Outport  Port=3
  Fz_c : Outport  Port=4
  Mx_c : Outport  Port=5
  My_c : Outport  Port=6
  Mz_c : Outport  Port=7
  wires:
  Constant8/1 -> Mux3/3
  Constant7/1 -> Mux3/2
  Peso/1 -> Monitor1/1, Gain1/1
  Matrix Concatenate/1 -> "[F,M]"/1  "Cambio Eje Z"
  Quaternion Rotation6/1 -> Display2/1, Ajuste  Momento/1, Matrix Concatenate/2
  Fuerzas1/1 -> Matrix Concatenate/1, Display10/1, Ajuste Fuerzas/1, Quaternion Rotation3/2
  Demux/1 -> Fx_c/1
  Demux/3 -> Fz_c/1
  Demux/2 -> Fy_c/1
  Demux1/2 -> My_c/1
  Demux1/1 -> Mx_c/1
  Demux1/3 -> Mz_c/1
  Constant9/1 -> Mux6/2
  Constant2/1 -> Mux6/1
  Gain1/1 -> Mux6/3
  Ajuste  Momento/1 -> Demux1/1
  Ajuste Fuerzas/1 -> Demux/1
  Quaternion de Giro (Ejes Globales a Cuerpo)/1 -> Display9/1, [Qgb]
  Quaternion de Giro (Ejes Viento a Cuerpo)/1 -> Display1/1, [Qvb]
  Mux5/1 -> Quaternion Rotation6/2
  My/1 -> Gain6/1
  Mx/1 -> Gain7/1
  Mz/1 -> Gain4/1
  Mux6/1 -> Quaternion Rotation5/2
  [Qgb] -> Quaternion Rotation5/1
  Trac/1 -> Monitor/1, Gain8/1
  Quaternion Rotation5/1 -> Fuerzas1/3
  Mux3/1 -> Fuerzas1/2
  Mux1/1 -> Quaternion Rotation7/2
  [Qvb] -> Quaternion Rotation7/1
  Quaternion Rotation7/1 -> Fuerzas1/1
  Gain2/1 -> Mux1/1
  Drag/1 -> Gain2/1
  SideForce/1 -> Gain3/1
  Lift/1 -> Gain5/1
  Quaternion Rotation3/1 -> Display6/1
  Quaternion Inverse/1 -> Quaternion Rotation3/1
  [Qvb] -> Quaternion Inverse/1
  [Qvb] -> Quaternion Rotation6/1
  Gain3/1 -> Mux1/2
  Gain4/1 -> Mux5/3
  Gain5/1 -> Mux1/3
  Gain6/1 -> Mux5/2
  Gain7/1 -> Mux5/1
  Gain8/1 -> Mux3/1

== system Mission__SimulatorModel/Matriz de Cambio de Ejes Globales a Cuerpo QUATERNIONES ==
  psi : Inport
  theta : Inport  Port=2
  phi : Inport  Port=3
  Angle Conversion7 : aerolibconvert2/Angle Conversion  IU=deg  OU=rad
  Coordinate Transformation Conversion : robotcorelib/Coordinate Transformation Conversion  InputRepresentation=Quaternion  InputEulerSequence=ZYX  ShowTrVecInputPort=on  OutputRepresentation=Rotation Matrix  OutputEulerSequence=ZYX  ShowTrVecOutputPort=on  SimulateUsing=Interpreted execution
      settings: SourceProductBaseCode=NV,RO,RR
  Rotation Angles to Quaternions1 : sharedtransform/Rotation Angles to Quaternions  rotationOrder=XYZ  aMode=aMode
      settings: SourceProductBaseCode=AE,PW,MT,VE,VP
  Vector Concatenate : Concatenate  NumInputs=3
  Matrix : Outport
  Quat : Outport  Port=2
  wires:
  Coordinate Transformation Conversion/1 -> Matrix/1
  phi/1 -> Vector Concatenate/1
  Angle Conversion7/1 -> Rotation Angles to Quaternions1/1
  Vector Concatenate/1 -> Angle Conversion7/1
  psi/1 -> Vector Concatenate/3
  theta/1 -> Vector Concatenate/2
  Rotation Angles to Quaternions1/1 -> Coordinate Transformation Conversion/1, Quat/1

== system Mission__SimulatorModel/Matriz de Cambio de Ejes Viento a Cuerpo QUATERNIONES ==
  xi : Inport
  gamma : Inport  Port=2
  mu : Inport  Port=3
  Angle Conversion7 : aerolibconvert2/Angle Conversion  IU=deg  OU=rad
  Coordinate Transformation Conversion : robotcorelib/Coordinate Transformation Conversion  InputRepresentation=Quaternion  InputEulerSequence=ZYX  ShowTrVecInputPort=on  OutputRepresentation=Rotation Matrix  OutputEulerSequence=ZYX  ShowTrVecOutputPort=on  SimulateUsing=Interpreted execution
      settings: SourceProductBaseCode=NV,RO,RR
  Rotation Angles to Quaternions1 : sharedtransform/Rotation Angles to Quaternions  rotationOrder=XYZ  aMode=aMode
      settings: SourceProductBaseCode=AE,PW,MT,VE,VP
  Vector Concatenate : Concatenate  NumInputs=3
  Matrix : Outport
  Quat : Outport  Port=2
  wires:
  Rotation Angles to Quaternions1/1 -> Quat/1, Coordinate Transformation Conversion/1
  gamma/1 -> Vector Concatenate/2
  xi/1 -> Vector Concatenate/3
  mu/1 -> Vector Concatenate/1
  Coordinate Transformation Conversion/1 -> Matrix/1
  Angle Conversion7/1 -> Rotation Angles to Quaternions1/1
  Vector Concatenate/1 -> Angle Conversion7/1

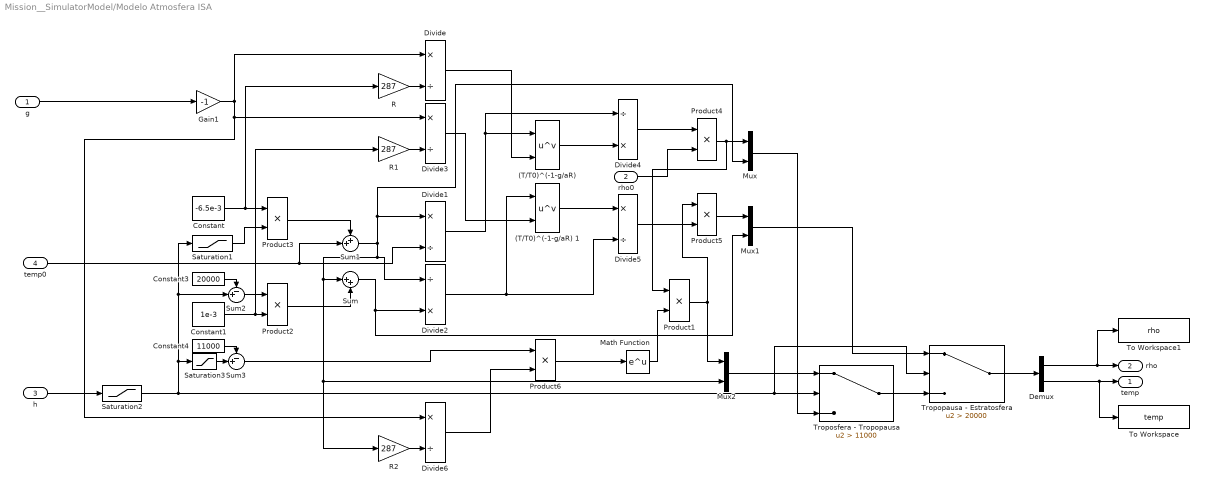
== system Mission__SimulatorModel/Modelo Atmosfera ISA ==
  g : Inport
  " rho0" : Inport  Port=2
  h : Inport  Port=3
  temp0 : Inport  Port=4
  "(T/T0)^(-1-g/aR) " : Math  Operator=pow  SignedPower=on  SaturateOnIntegerOverflow=on
  (T/T0)^(-1-g/aR) 1 : Math  Operator=pow  SignedPower=on  SaturateOnIntegerOverflow=on
  Constant : Constant  Value=-6.5e-3
  Constant1 : Constant  Value=1e-3
  Constant3 : Constant  Value=20000
  Constant4 : Constant  Value=11000
  Demux : Demux  Outputs=2
  Divide{,1,3,5..6} (5 alike) : Product  Inputs=*/
  Divide2 : Product  Inputs=/*
  Divide4 : Product  Inputs=/*
  Gain1 : Gain  Gain=-1
  Math Function : Math  SaturateOnIntegerOverflow=on
  Mux : Mux  Inputs=2
  Mux1 : Mux  Inputs=2
  Mux2 : Mux  Inputs=2
  Product{1..6} (6 alike) : Product
  R : Gain  Gain=287
  R1 : Gain  Gain=287
  R2 : Gain  Gain=287
  Saturation1 : Saturate  UpperLimit=11000  LowerLimit=0
  Saturation2 : Saturate  UpperLimit=32000  LowerLimit=0
  Saturation3 : Saturate  UpperLimit=20000  LowerLimit=0
  Sum : Sum  Inputs=|++
  Sum1 : Sum  Inputs=++|
  Sum2 : Sum  Inputs=-+|
  Sum3 : Sum  Inputs=-+|
  To Workspace : ToWorkspace  VariableName=temp  SampleTime=-1
  To Workspace1 : ToWorkspace  VariableName=rho  SampleTime=-1
  Tropopausa - Estratosfera : Switch  Criteria=u2 > Threshold  Threshold=20000
  Troposfera - Tropopausa : Switch  Criteria=u2 > Threshold  Threshold=11000
  temp : Outport
  rho : Outport  Port=2
  wires:
  R/1 -> Divide/2
  Gain1/1 -> Divide3/1, Divide6/1, Divide/1
  g/1 -> Gain1/1
  Troposfera - Tropopausa/1 -> Tropopausa - Estratosfera/3
  h/1 -> Saturation2/1
  temp0/1 -> Divide1/2, Sum1/2
  Constant/1 -> Product3/1, R/1
  Constant1/1 -> R1/1, Product2/2
  Product3/1 -> Sum1/1
  Sum/1 -> Mux1/2, Divide2/2
  Sum1/1 -> Divide2/1, Mux2/2, R2/1, Sum/1, Mux/2, Divide1/1
  R1/1 -> Divide3/2
  Divide1/1 -> Divide4/1, "(T/T0)^(-1-g/aR) "/1
  Divide/1 -> "(T/T0)^(-1-g/aR) "/2
  Divide3/1 -> (T/T0)^(-1-g/aR) 1/2
  Divide2/1 -> (T/T0)^(-1-g/aR) 1/1, Divide5/2
  (T/T0)^(-1-g/aR) 1/1 -> Divide5/1
  "(T/T0)^(-1-g/aR) "/1 -> Divide4/2
  Divide4/1 -> Product4/1
  Divide5/1 -> Product5/2
  " rho0"/1 -> Product4/2
  Product4/1 -> Product1/1, Mux/1
  Product5/1 -> Mux1/1
  Product2/1 -> Sum/2
  Saturation1/1 -> Product3/2
  Sum2/1 -> Product2/1
  Constant3/1 -> Sum2/1
  Mux/1 -> Troposfera - Tropopausa/3
  Mux1/1 -> Tropopausa - Estratosfera/1
  Tropopausa - Estratosfera/1 -> Demux/1
  Demux/1 -> To Workspace1/1, rho/1
  Demux/2 -> To Workspace/1, temp/1
  Mux2/1 -> Troposfera - Tropopausa/1
  Product1/1 -> Product5/1, Mux2/1
  Math Function/1 -> Product1/2
  Constant4/1 -> Sum3/1
  R2/1 -> Divide6/2
  Product6/1 -> Math Function/1
  Sum3/1 -> Product6/1
  Divide6/1 -> Product6/2
  Saturation2/1 -> Saturation3/1, Sum2/2, Saturation1/1, Troposfera - Tropopausa/2, Tropopausa - Estratosfera/2
  Saturation3/1 -> Sum3/2

== system Mission__SimulatorModel/Normal1 ==
  x : Inport
  y : Inport  Port=2
  Abs : Abs
  Abs1 : Abs
  Add8 : Sum
  Derivative : Derivative
  Derivative1 : Derivative
  Integrator : Integrator
  Integrator1 : Integrator
  Product4 : Product
  Product5 : Product
  Sqrt : Sqrt  SaturateOnIntegerOverflow=on
  |Acumulative Distance| : Outport
  wires:
  Product5/1 -> Add8/2
  Product4/1 -> Add8/1
  Add8/1 -> Sqrt/1
  x/1 -> Derivative/1
  y/1 -> Derivative1/1
  Derivative/1 -> Abs/1
  Derivative1/1 -> Abs1/1
  Abs/1 -> Integrator/1
  Abs1/1 -> Integrator1/1
  Integrator1/1 -> Product5/1, Product5/2
  Integrator/1 -> Product4/2, Product4/1
  Sqrt/1 -> |Acumulative Distance|/1

== system Mission__SimulatorModel/Subsystem q ==
  rho : Inport
  V : Inport  Port=2
  " Velocidad" : Display
  Gain : Gain  Gain=0.5
  Math Function : Math  Operator=square  SaturateOnIntegerOverflow=on
  Product : Product
  q : Outport
  wires:
  Gain/1 -> Product/2
  Product/1 -> q/1  "q"
  V/1 -> Math Function/1, " Velocidad"/1
  rho/1 -> Product/1
  Math Function/1 -> Gain/1

== system Mission__SimulatorModel/Subsystem10 ==
  Altura : Inport
  Fz : Inport  Port=2
  Constant7 : Constant  Value=0
  Switch5 : Switch  Criteria=u2 > Threshold
  Switch6 : Switch
  Fz con Suelo : Outport
  wires:
  Altura/1 -> Switch5/2
  Fz/1 -> Switch6/2, Switch5/1, Switch6/1
  Switch5/1 -> Fz con Suelo/1
  Constant7/1 -> Switch6/3
  Switch6/1 -> Switch5/3

== system Mission__SimulatorModel/Subsystem11 ==
  Vz : Inport
  Altura : Inport  Port=2
  Constant7 : Constant  Value=0
  Switch5 : Switch
  Switch6 : Switch
  Vz con Suelo : Outport
  wires:
  Altura/1 -> Switch5/2
  Vz/1 -> Switch5/1, Switch6/2, Switch6/1
  Switch5/1 -> Vz con Suelo/1
  Constant7/1 -> Switch6/3
  Switch6/1 -> Switch5/3

== system Mission__SimulatorModel/Subsystem12 ==
  Altura : Inport
  Vz : Inport  Port=2
  Constant7 : Constant  Value=0
  Switch5 : Switch  Criteria=u2 > Threshold
  Switch6 : Switch
  Vz con Suelo : Outport
  wires:
  Altura/1 -> Switch5/2
  Vz/1 -> Switch5/1, Switch6/2, Switch6/1
  Switch5/1 -> Vz con Suelo/1
  Constant7/1 -> Switch6/3
  Switch6/1 -> Switch5/3

== system Mission__SimulatorModel/Subsystem13 ==
  Altura : Inport
  My : Inport  Port=2
  theta : Inport  Port=3
  Saturation : Saturate  UpperLimit=inf  LowerLimit=0
  Switch5 : Switch  Criteria=u2 > Threshold
  Switch6 : Switch  Criteria=u2 > Threshold
  My con Suelo : Outport
  wires:
  Switch6/1 -> Switch5/3
  Saturation/1 -> Switch6/3
  My/1 -> Saturation/1, Switch6/1, Switch5/1
  Altura/1 -> Switch5/2
  theta/1 -> Switch6/2
  Switch5/1 -> My con Suelo/1

== system Mission__SimulatorModel/Subsystem14 ==
  Altura : Inport
  theta : Inport  Port=2
  Constant7 : Constant  Value=0
  Switch5 : Switch  Criteria=u2 > Threshold
  Switch6 : Switch
  theta con Suelo : Outport
  wires:
  Switch6/1 -> Switch5/3
  Constant7/1 -> Switch6/3
  theta/1 -> Switch6/1, Switch6/2, Switch5/1
  Altura/1 -> Switch5/2
  Switch5/1 -> theta con Suelo/1

== system Mission__SimulatorModel/Subsystem15 ==
  IAS : Inport
  h : Inport  Port=2
  Distance : Inport  Port=3
  Clock : Clock
  Constant : Constant
  Constant1 : Constant  Value=Mission_Data
  Constant2 : Constant  Value=psi_ini
  Constant4 : Constant  Value=0
  Constant8 : Constant  Value=Mission
  Delay1 : Delay  DelayLength=1  InitialCondition=0
  Delay2 : Delay  DelayLength=1  InitialCondition=0
  Jump Limiter : Subsystem
  MATLAB Function : MATLAB Function  TreatAsAtomicUnit=on
  Mux1 : Mux  Inputs=3
  Mux2 : Mux
  Mux8 : Mux  Inputs=3
  Saturation : Saturate  UpperLimit=length(Mission_Data(:,1))+1  LowerLimit=0
  Scope : Scope  NumInputPorts=2
  Signal Restarter : Subsystem
      settings: PortSchema="{\"entries\":[{\"content\":{\"sides\":[{\"content\":{\"connectorIds\":[\"In1\"]},\"type\":\"ConnectorPlacement.EquallySpacedRectSide\",\"uuid\":\"aa7cd995-5add-4439-b75e-9bd33f63979b\"},{\"content\":{\"connectorIds\":[\"Out1\"],\"side\":\"RIGHT\"},\"type\":\"ConnectorPlacement.EquallySpacedRectSide\",\"uuid\":\"0a676ad3-7f96-4bdf-b2c7-7ebf31bab36a\"},{\"content\":{\"connectorIds\":[\"In2\"],\"side\":\"TOP\"},\"type\":\"ConnectorPlacement.EquallySpacedRectSide\",\"uuid\":\"608e60f9-c604-4d4a-9d82-45bcdebed7ae\"}]},\"type\":\"ConnectorPlacement.EquallySpacedConnector\",\"uuid\":\"c2af05c1-165b-41b6-9cdb-7d75cabff9ea\"}],\"packageUris\":[\"http://schema.mathworks.com/mf0/Connector/19700101\"],\"version\":\"1.0\"}"
  Stop Simulation : Stop
  Sum : Sum  Inputs=+++
  Switch1 : Switch  Criteria=u2 ~= 0  Threshold=5
  Autopilot : Outport
  Mission ON/OFF : Outport  Port=2
  Autopilot ON/OF : Outport  Port=3
  wires:
  Constant8/1 -> Mission ON/OFF/1
  Constant1/1 -> MATLAB Function/1(OpData)
  IAS/1 -> Mux1/1
  h/1 -> Mux1/2
  Mux1/1 -> MATLAB Function/3(StateData)
  MATLAB Function/4(c0) -> Mux2/1
  MATLAB Function/7(c_hdg) -> Mux2/4
  MATLAB Function/6(c_vel) -> Mux2/3
  MATLAB Function/5(c_alt) -> Mux2/2
  MATLAB Function/3(d3) -> Mux8/3
  MATLAB Function/1(d1) -> Mux8/1
  MATLAB Function/2(d2) -> Mux8/2
  Mux8/1 -> Autopilot/1
  Mux2/1 -> Autopilot ON/OF/1
  MATLAB Function/8(stop) -> Stop Simulation/1
  Distance/1 -> Signal Restarter/1(Full Signal)
  Signal Restarter/1(Trunked Signal) -> Mux1/3
  Constant2/1 -> MATLAB Function/4(psi_ini)
  Constant/1 -> Switch1/3
  Constant4/1 -> Switch1/1
  Clock/1 -> Switch1/2
  Switch1/1 -> Sum/2
  Delay2/1 -> Sum/1
  Delay1/1 -> Scope/2, Sum/3
  MATLAB Function/9(next) -> Delay1/1
  Saturation/1 -> Signal Restarter/2(Index), MATLAB Function/2(Index)
  Sum/1 -> Jump Limiter/1("Input ")
  Jump Limiter/1(Output Limited) -> Scope/1, Saturation/1, Delay2/1

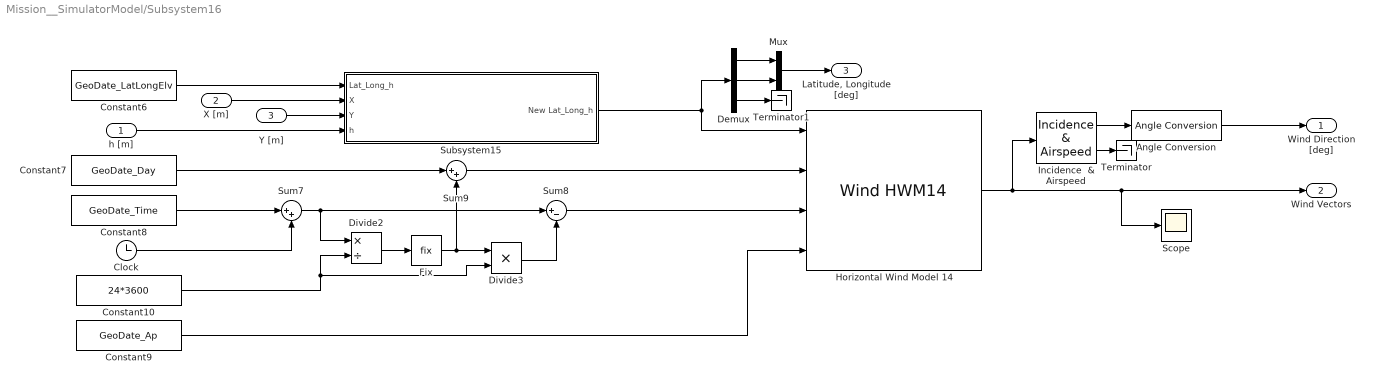
== system Mission__SimulatorModel/Subsystem16 ==
  h [m] : Inport
  X [m] : Inport  Port=2
  Y [m] : Inport  Port=3
  Angle Conversion : aerolibconvert2/Angle Conversion  IU=rad  OU=deg
  Clock : Clock
  Constant10 : Constant  Value=24*3600
  Constant6 : Constant  Value=GeoDate_LatLongElv
  Constant7 : Constant  Value=GeoDate_Day
  Constant8 : Constant  Value=GeoDate_Time
  Constant9 : Constant  Value=GeoDate_Ap
  Demux : Demux  Outputs=3
  Divide2 : Product  Inputs=*/
  Divide3 : Product  Inputs=**
  Fix : Rounding  Operator=fix
  Horizontal Wind Model 14 : WindHWM14  model=Total
  Incidence  & Airspeed : aerolibasang/Incidence  & Airspeed
      settings: SourceProductBaseCode=AE
  Mux : Mux  Inputs=2
  Scope : Scope
  Subsystem15 : Subsystem
  Sum7 : Sum  Inputs=|++
  Sum8 : Sum  Inputs=|+-
  Sum9 : Sum  Inputs=|++
  Terminator : Terminator
  Terminator1 : Terminator
  Wind Direction [deg] : Outport
  Wind Vectors : Outport  Port=2
  "Latitude, Longitude [deg]" : Outport  Port=3
  wires:
  Fix/1 -> Divide3/1, Sum9/2
  Sum8/1 -> Horizontal Wind Model 14/3
  Clock/1 -> Sum7/2
  Constant10/1 -> Divide3/2, Divide2/2
  Constant9/1 -> Horizontal Wind Model 14/4
  Constant7/1 -> Sum9/1
  Horizontal Wind Model 14/1 -> Scope/1, Wind Vectors/1, Incidence  & Airspeed/1
  Constant8/1 -> Sum7/1
  Sum9/1 -> Horizontal Wind Model 14/2
  Divide2/1 -> Fix/1
  Divide3/1 -> Sum8/2
  Sum7/1 -> Sum8/1, Divide2/1
  h [m]/1 -> Subsystem15/4(h)
  Incidence  & Airspeed/2 -> Terminator/1
  Incidence  & Airspeed/1 -> Angle Conversion/1
  Angle Conversion/1 -> Wind Direction [deg]/1
  Subsystem15/1(New Lat_Long_h) -> Demux/1, Horizontal Wind Model 14/1
  Constant6/1 -> Subsystem15/1(Lat_Long_h)
  X [m]/1 -> Subsystem15/2(X)
  Y [m]/1 -> Subsystem15/3(Y)
  Demux/3 -> Terminator1/1
  Demux/1 -> Mux/1
  Demux/2 -> Mux/2
  Mux/1 -> "Latitude, Longitude [deg]"/1

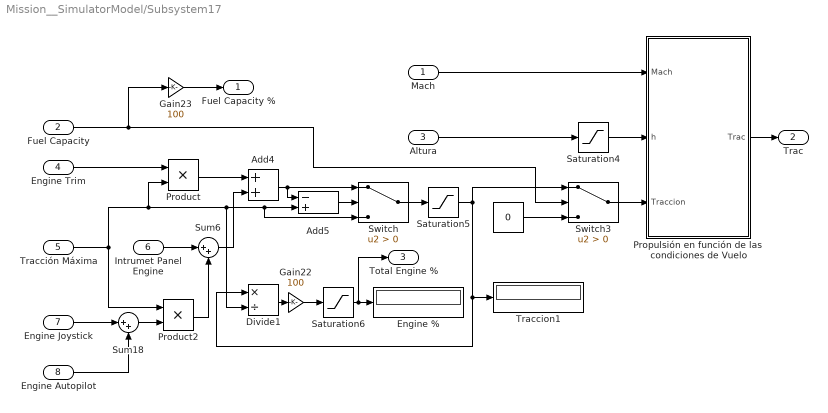
== system Mission__SimulatorModel/Subsystem17 ==
  Mach : Inport
  Fuel Capacity : Inport  Port=2
  Altura : Inport  Port=3
  Engine Trim : Inport  Port=4
  Tracción Máxima : Inport  Port=5
  Intrumet Panel Engine : Inport  Port=6
  Engine Joystick : Inport  Port=7
  Engine Autopilot : Inport  Port=8
  "                       " : Constant  Value=0
  Add4 : Sum
  Add5 : Sum  Inputs=-+
  Divide1 : Product  Inputs=*/
  Engine % : Display
  Gain22 : Gain  Gain=100
  Gain23 : Gain  Gain=100
  Product : Product
  Product2 : Product
  Propulsión en función de las  condiciones de Vuelo : Subsystem
  Saturation4 : Saturate  UpperLimit=OperativeCeiling  LowerLimit=0
  Saturation5 : Saturate  UpperLimit=inf  LowerLimit=0
  Saturation6 : Saturate  UpperLimit=inf  LowerLimit=-20
  Sum18 : Sum  Inputs=|++
  Sum6 : Sum  Inputs=|++
  Switch : Switch  Criteria=u2 > Threshold
  Switch3 : Switch  Criteria=u2 > Threshold
  Traccion1 : Display
  Fuel Capacity % : Outport
  Trac : Outport  Port=2
  Total Engine % : Outport  Port=3
  wires:
  Product/1 -> Add4/1
  Altura/1 -> Saturation4/1
  Saturation4/1 -> Propulsión en función de las  condiciones de Vuelo/2(h)
  Sum18/1 -> Product2/2
  Divide1/1 -> Gain22/1
  Switch/1 -> Saturation5/1
  Propulsión en función de las  condiciones de Vuelo/1(Trac) -> Trac/1
  Add4/1 -> Add5/1, Switch/1
  Saturation5/1 -> Switch3/1, Divide1/1, Traccion1/1
  Gain23/1 -> Fuel Capacity %/1
  Switch3/1 -> Propulsión en función de las  condiciones de Vuelo/3(Traccion)
  Sum6/1 -> Add4/2
  Product2/1 -> Sum6/2
  Fuel Capacity/1 -> Gain23/1, Switch3/2
  Gain22/1 -> Saturation6/1
  Engine Joystick/1 -> Sum18/1
  Add5/1 -> Switch/2
  "                       "/1 -> Switch3/3
  Saturation6/1 -> Total Engine %/1, Engine %/1
  Mach/1 -> Propulsión en función de las  condiciones de Vuelo/1(Mach)
  Engine Trim/1 -> Product/1
  Intrumet Panel Engine/1 -> Sum6/1
  Tracción Máxima/1 -> Product2/1, Product/2, Divide1/2, Switch/3, Add5/2
  Engine Autopilot/1 -> Sum18/2
